simulink model "CoESS_Dem"  (R2016b)
settings: configuration reference "CodeGenConfigSet" (kept outside this file)
values from neighbouring files (symbols this model uses):
  ESS_nMax_C = Calibration.Parameter    [init_CoESS_Dem.m]
  ESS_nMin_C = Calibration.Parameter    [init_CoESS_Dem.m]
  ESS_trqDesAcs_C = Calibration.Parameter    [init_CoESS_Dem.m]
  ESS_trqResvAcs_C = Calibration.Parameter    [init_CoESS_Dem.m]
settings Model: Creator=Wollf  LastModifiedBy=lenovo
settings ConfigSetRef: SourceLocation=Base Workspace

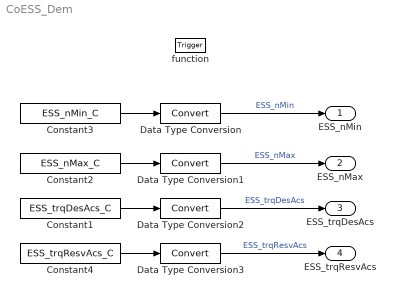
== system CoESS_Dem ==
  function : TriggerPort  TriggerType=function-call  VariantControl=Variant
  Constant1 : Constant  Value=ESS_trqDesAcs_C
  Constant2 : Constant  Value=ESS_nMax_C
  Constant3 : Constant  Value=ESS_nMin_C
  Constant4 : Constant  Value=ESS_trqResvAcs_C
  Data Type Conversion{,1..3} (4 alike) : DataTypeConversion
  ESS_nMin : Outport  Tag=rpm  Description=Min. engine speed request from Electrical Supply System  OutMin=-6000  OutMax=6000  OutDataTypeStr=EngSpeed_rpm
  ESS_nMax : Outport  Tag=rpm  Description=Max. engine speed request from Electrical Supply System  Port=2  OutMin=-6000  OutMax=6000  OutDataTypeStr=EngSpeed_rpm
  ESS_trqDesAcs : Outport  Tag=Nm  Description=Torque request from Electrical Supply System  Port=3  OutMin=-3000  OutMax=3276.7  OutDataTypeStr=Trq_Nm
  ESS_trqResvAcs : Outport  Tag=Nm  Description=Torque reserve due to on-board electrical system  Port=4  OutMin=-3000  OutMax=3276.7  OutDataTypeStr=Trq_Nm
  wires:
  Constant3/1 -> Data Type Conversion/1
  Constant2/1 -> Data Type Conversion1/1
  Constant1/1 -> Data Type Conversion2/1
  Constant4/1 -> Data Type Conversion3/1
  Data Type Conversion/1 -> ESS_nMin/1  "ESS_nMin"
  Data Type Conversion1/1 -> ESS_nMax/1  "ESS_nMax"
  Data Type Conversion2/1 -> ESS_trqDesAcs/1  "ESS_trqDesAcs"
  Data Type Conversion3/1 -> ESS_trqResvAcs/1  "ESS_trqResvAcs"
